simulink model "sampleModel1990"  (R2023a)
settings: Solver=VariableStepAuto  StartTime=0.0  StopTime=10.0  RelTol=1e-3
libraries: hdlsllib x1, simulink x1
settings Model: Creator=user1  LastModifiedBy=user1

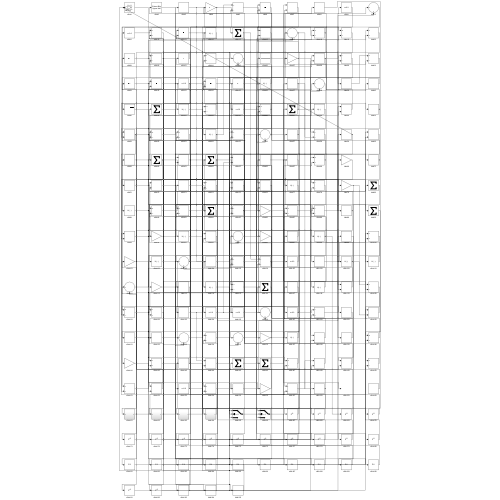
[thumbnail: Simulink's stored preview of the top-level diagram]
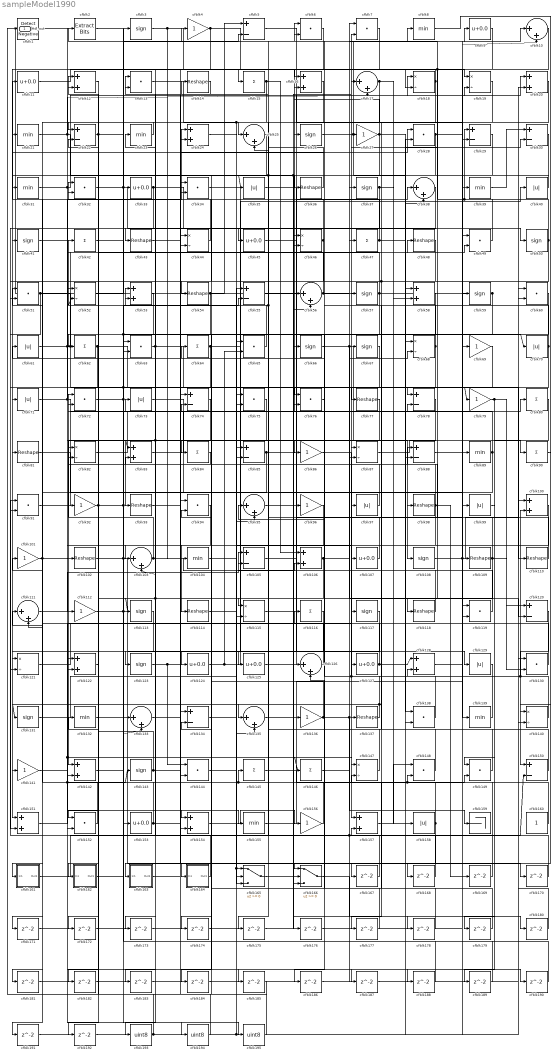
== system sampleModel1990 ==
  cfblk1 : hdlsllib/Logic and Bit Operations/Detect Fall Negative  vinit=0  OutDataTypeStr=uint8
  cfblk{10,17,25,38,56,95,103,111,126,133,135} (11 alike) : Sum  Inputs=|++  OutDataTypeStr=uint8
  cfblk{12,16,20,24,53,58,83,100,106,122,128,142,151,154,157} (15 alike) : Sum  OutDataTypeStr=uint8
  cfblk{4,27,69,79,86,92,96,101,112,136,141,156} (12 alike) : Gain  OutDataTypeStr=uint8
  cfblk{14,36,43,48,54,77,81,93,98,102,109..110,114,118,137} (15 alike) : Reshape
  cfblk{8,21,23,31,39,89,104,132,139,155} (10 alike) : MinMax  OutDataTypeStr=uint8
  cfblk{5,22,29..30,55,74,78,85,88,105,120,134,150} (13 alike) : Sum  Inputs=+-  OutDataTypeStr=uint8
  cfblk{9,11,33,45,107,124..125,127,153} (9 alike) : Bias  Bias=0.0  SaturateOnIntegerOverflow=off
  cfblk{3,26,37,41,50,57,59,66..67,108,113,117,123,131,143} (15 alike) : Signum
  cfblk{18..19,44,46,52,68,82,87,115,121,140,147} (12 alike) : Product  Inputs=*/  OutDataTypeStr=uint8  RndMeth=Zero  SaturateOnIntegerOverflow=on
  cfblk{15,42,47,62,64,80,84,90,116,145..146} (11 alike) : Sum  Inputs=+  OutDataTypeStr=uint8
  cfblk{6..7,13,28,32,34,49,51,60,63,65,72,75..76,91,94,119,130,138,144,148..149,152} (23 alike) : DotProduct  OutDataTypeStr=uint8
  cfblk{35,40,61,70..71,73,97,99,129,158} (10 alike) : Abs  OutDataTypeStr=uint8  SaturateOnIntegerOverflow=off
  cfblk159 : Terminator
  cfblk160 : Constant  OutDataTypeStr=uint8  SampleTime=-1
  cfblk161 : Subsystem
      settings: LibrarySourceBlock=|
      | hdlsllib/Ports &
      | Subsystems/Subsystem
  cfblk162 : Subsystem
      settings: LibrarySourceBlock=|
      | hdlsllib/Ports &
      | Subsystems/Subsystem
  cfblk163 : Subsystem
      settings: LibrarySourceBlock=|
      | hdlsllib/Ports &
      | Subsystems/Subsystem
  cfblk164 : Subsystem
      settings: LibrarySourceBlock=|
      | hdlsllib/Ports &
      | Subsystems/Subsystem
  cfblk165 : Switch  OutDataTypeStr=uint8  SaturateOnIntegerOverflow=off  InputSameDT=off
  cfblk166 : Switch  OutDataTypeStr=uint8  SaturateOnIntegerOverflow=off  InputSameDT=off
  cfblk{167..192} (26 alike) : Delay  SampleTime=1
  cfblk193 : DataTypeConversion  OutDataTypeStr=uint8  SaturateOnIntegerOverflow=off  RndMeth=Floor
  cfblk194 : DataTypeConversion  OutDataTypeStr=uint8  SaturateOnIntegerOverflow=off  RndMeth=Floor
  cfblk195 : DataTypeConversion  OutDataTypeStr=uint8  SaturateOnIntegerOverflow=off  RndMeth=Floor
  cfblk2 : simulink/Logic and Bit Operations/Extract Bits  bitsToExtract=Upper half  numBits=8  bitIdxRange=[0 7]  outScalingMode=Preserve fixed-point scaling
      settings: LibrarySourceBlock=|
      | hdlsllib/Logic and Bit
      | Operations/Extract Bits
  Hdl_out : Outport  OutDataTypeStr=uint8
  wires:
  cfblk103/1 -> cfblk72/1, cfblk106/2
  cfblk95/1 -> cfblk18/1
  cfblk4/1 -> cfblk151/1, cfblk39/1
  cfblk65/1 -> cfblk42/1
  cfblk157/1 -> cfblk148/1
  cfblk160/1 -> cfblk148/2, cfblk53/2
  cfblk116/1 -> cfblk161/1(In1)
  cfblk64/1 -> cfblk141/1, cfblk110/1
  cfblk57/1 -> cfblk135/1, cfblk6/2
  cfblk82/1 -> cfblk19/1
  cfblk15/1 -> cfblk25/1, cfblk106/1
  cfblk14/1 -> cfblk13/1
  cfblk86/1 -> cfblk157/1
  cfblk123/1 -> cfblk144/1, cfblk48/1
  cfblk46/1 -> cfblk26/1, cfblk51/2
  cfblk49/1 -> cfblk29/1, cfblk4/1
  cfblk139/1 -> cfblk7/2
  cfblk153/1 -> cfblk101/1, cfblk165/2
  cfblk138/1 -> cfblk87/1, cfblk95/1
  cfblk125/1 -> cfblk38/1
  cfblk75/1 -> cfblk93/1
  cfblk24/1 -> cfblk107/1
  cfblk45/1 -> cfblk127/1
  cfblk34/1 -> cfblk129/1
  cfblk69/1 -> cfblk78/1
  cfblk77/1 -> cfblk142/1
  cfblk91/1 -> cfblk73/1
  cfblk71/1 -> cfblk78/2, cfblk34/1
  cfblk143/1 -> cfblk12/1, cfblk170/1
  cfblk158/1 -> cfblk111/2, cfblk173/1
  cfblk62/1 -> cfblk76/1, cfblk121/1
  cfblk31/1 -> cfblk146/1, cfblk187/1, cfblk19/2
  cfblk148/1 -> cfblk57/1
  cfblk38/1 -> cfblk91/2
  cfblk26/1 -> cfblk9/1, cfblk138/1
  cfblk48/1 -> cfblk102/1
  cfblk137/1 -> cfblk131/1, cfblk72/2
  cfblk124/1 -> cfblk40/1, cfblk65/2
  cfblk121/1 -> cfblk117/1
  cfblk23/1 -> cfblk22/1
  cfblk1/1 -> cfblk112/1
  cfblk8/1 -> cfblk166/1
  cfblk109/1 -> cfblk152/1, cfblk88/1, cfblk130/2
  cfblk101/1 -> cfblk154/1, cfblk31/1
  cfblk119/1 -> cfblk105/1
  cfblk163/1(Out1) -> cfblk44/1
  cfblk102/1 -> cfblk166/2, cfblk195/1
  cfblk53/1 -> cfblk122/1
  cfblk130/1 -> cfblk66/1
  cfblk127/1 -> cfblk128/1, cfblk52/1
  cfblk164/1(Out1) -> cfblk13/2
  cfblk74/1 -> cfblk92/1
  cfblk47/1 -> cfblk24/1, cfblk30/2
  cfblk42/1 -> cfblk79/1, cfblk185/1
  cfblk28/1 -> cfblk125/1, cfblk166/3, cfblk10/1
  cfblk55/1 -> cfblk126/1
  cfblk120/1 -> cfblk150/1
  cfblk39/1 -> cfblk30/1
  cfblk146/1 -> cfblk47/1
  cfblk128/1 -> cfblk69/1
  cfblk25/1 -> cfblk81/1
  cfblk134/1 -> cfblk147/1
  cfblk35/1 -> cfblk89/1
  cfblk22/1 -> cfblk62/1, cfblk190/1
  cfblk13/1 -> cfblk135/2
  cfblk129/1 -> cfblk128/2
  cfblk66/1 -> cfblk108/1, cfblk119/2
  cfblk73/1 -> cfblk139/1
  cfblk33/1 -> cfblk95/2, cfblk192/1
  cfblk107/1 -> cfblk53/1
  cfblk9/1 -> cfblk71/1
  cfblk149/1 -> cfblk32/1
  cfblk92/1 -> cfblk153/1, cfblk55/2, cfblk22/2, cfblk162/1(In1)
  cfblk40/1 -> cfblk36/1
  cfblk63/1 -> cfblk96/1, cfblk103/1
  cfblk97/1 -> cfblk23/1
  cfblk161/1(Out1) -> cfblk150/2, cfblk67/1
  cfblk6/1 -> cfblk113/1, cfblk183/1
  cfblk83/1 -> cfblk37/1
  cfblk36/1 -> cfblk14/1
  cfblk44/1 -> cfblk11/1
  cfblk60/1 -> cfblk123/1
  cfblk5/1 -> cfblk119/1
  cfblk100/1 -> cfblk137/1
  cfblk88/1 -> cfblk80/1
  cfblk151/1 -> cfblk143/1, cfblk116/1
  cfblk51/1 -> cfblk134/1, cfblk121/2
  cfblk78/1 -> cfblk84/1
  cfblk87/1 -> cfblk90/1
  cfblk81/1 -> cfblk133/1
  cfblk93/1 -> cfblk20/1
  cfblk41/1 -> cfblk49/2
  cfblk68/1 -> cfblk163/1(In1), cfblk24/2
  cfblk7/1 -> cfblk83/1, cfblk103/2
  cfblk12/1 -> cfblk82/1
  cfblk67/1 -> cfblk122/2
  cfblk140/1 -> cfblk100/2, cfblk61/1
  cfblk133/1 -> cfblk28/1
  cfblk21/1 -> cfblk56/2, cfblk17/2
  cfblk147/1 -> cfblk2/1
  cfblk11/1 -> cfblk15/1
  cfblk136/1 -> cfblk68/2, cfblk159/1, cfblk64/1
  cfblk10/1 -> cfblk154/2, cfblk118/1
  cfblk54/1 -> cfblk63/2, cfblk5/1
  cfblk155/1 -> cfblk99/1
  cfblk30/1 -> cfblk54/1
  cfblk37/1 -> cfblk41/1, cfblk58/2
  cfblk156/1 -> cfblk145/1, cfblk34/2
  cfblk105/1 -> cfblk59/1
  cfblk29/1 -> cfblk35/1, cfblk45/1
  cfblk52/1 -> cfblk3/1
  cfblk2/1 -> cfblk98/1, cfblk70/1
  cfblk104/1 -> cfblk75/2
  cfblk154/1 -> cfblk156/1
  cfblk90/1 -> cfblk140/1
  cfblk79/1 -> cfblk149/1, cfblk120/1
  cfblk144/1 -> cfblk55/1
  cfblk70/1 -> cfblk151/2, cfblk6/1
  cfblk98/1 -> cfblk114/1, cfblk12/2, cfblk169/1
  cfblk145/1 -> cfblk149/2
  cfblk18/1 -> cfblk43/1, cfblk165/3, cfblk16/1
  cfblk108/1 -> cfblk20/2, cfblk10/2
  cfblk85/1 -> cfblk60/2, cfblk191/1
  cfblk162/1(Out1) -> cfblk157/2
  cfblk94/1 -> cfblk193/1
  cfblk84/1 -> cfblk82/2
  cfblk32/1 -> cfblk50/1, cfblk5/2
  cfblk3/1 -> cfblk18/2, cfblk104/1
  cfblk56/1 -> cfblk32/2, cfblk8/1
  cfblk112/1 -> cfblk136/1, cfblk133/2
  cfblk96/1 -> cfblk142/2
  cfblk131/1 -> cfblk85/2
  cfblk27/1 -> cfblk58/1, cfblk16/2, cfblk115/2
  cfblk126/1 -> cfblk51/1
  cfblk118/1 -> cfblk76/2
  cfblk132/1 -> cfblk74/2
  cfblk150/1 -> cfblk21/1, cfblk52/2
  cfblk152/1 -> cfblk111/1
  cfblk43/1 -> cfblk155/1
  cfblk58/1 -> cfblk164/1(In1)
  cfblk50/1 -> cfblk171/1, cfblk177/1, cfblk27/1
  cfblk72/1 -> cfblk77/1, cfblk88/2
  cfblk61/1 -> cfblk33/1, cfblk109/1, cfblk86/1
  cfblk89/1 -> cfblk46/2, cfblk115/1
  cfblk135/1 -> cfblk17/1
  cfblk106/1 -> cfblk124/1, cfblk120/2
  cfblk111/1 -> cfblk105/2
  cfblk17/1 -> cfblk158/1, cfblk172/1
  cfblk110/1 -> cfblk97/1
  cfblk113/1 -> cfblk152/2
  cfblk19/1 -> cfblk167/1
  cfblk167/1 -> cfblk46/1
  cfblk114/1 -> cfblk168/1
  cfblk168/1 -> cfblk25/2
  cfblk169/1 -> cfblk83/2
  cfblk170/1 -> cfblk91/1
  cfblk171/1 -> cfblk144/2
  cfblk172/1 -> cfblk28/2
  cfblk173/1 -> cfblk68/1
  cfblk59/1 -> cfblk174/1, Hdl_out/1
  cfblk174/1 -> cfblk56/1
  cfblk16/1 -> cfblk175/1
  cfblk175/1 -> cfblk7/1
  cfblk115/1 -> cfblk176/1
  cfblk176/1 -> cfblk29/2
  cfblk177/1 -> cfblk134/2
  cfblk166/1 -> cfblk178/1
  cfblk178/1 -> cfblk126/2
  cfblk99/1 -> cfblk179/1
  cfblk179/1 -> cfblk147/2
  cfblk165/1 -> cfblk180/1
  cfblk180/1 -> cfblk60/1
  cfblk20/1 -> cfblk181/1
  cfblk181/1 -> cfblk75/1
  cfblk122/1 -> cfblk182/1
  cfblk182/1 -> cfblk87/2
  cfblk183/1 -> cfblk44/2
  cfblk117/1 -> cfblk184/1
  cfblk184/1 -> cfblk38/2
  cfblk185/1 -> cfblk1/1
  cfblk76/1 -> cfblk186/1
  cfblk186/1 -> cfblk100/1
  cfblk187/1 -> cfblk140/2
  cfblk142/1 -> cfblk188/1
  cfblk188/1 -> cfblk63/1
  cfblk80/1 -> cfblk189/1
  cfblk189/1 -> cfblk74/1
  cfblk190/1 -> cfblk85/1
  cfblk191/1 -> cfblk138/2
  cfblk192/1 -> cfblk49/1
  cfblk193/1 -> cfblk165/1, cfblk65/1, cfblk130/1, cfblk132/1
  cfblk141/1 -> cfblk194/1
  cfblk194/1 -> cfblk94/1
  cfblk195/1 -> cfblk94/2

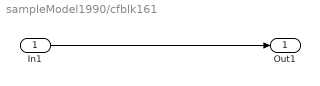
== system sampleModel1990/cfblk161 ==
  In1 : Inport
  Out1 : Outport
  wires:
  In1/1 -> Out1/1

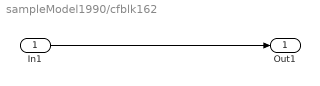
== system sampleModel1990/cfblk162 ==
  In1 : Inport
  Out1 : Outport
  wires:
  In1/1 -> Out1/1

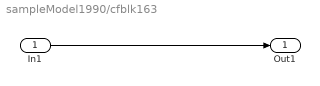
== system sampleModel1990/cfblk163 ==
  In1 : Inport
  Out1 : Outport
  wires:
  In1/1 -> Out1/1

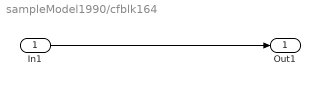
== system sampleModel1990/cfblk164 ==
  In1 : Inport
  Out1 : Outport
  wires:
  In1/1 -> Out1/1
